simulink subsystem "Leds"  (R2023b)
settings: Solver=VariableStepAuto  StartTime=0.0  StopTime=10.0  RelTol=1e-3
libraries: arduinolib x3
settings Model: Creator=Usuario_UMA  LastModifiedBy=Felix

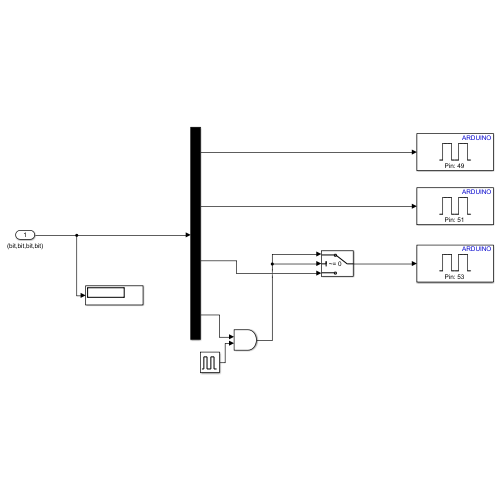
[thumbnail: Simulink's stored preview of the top-level diagram]
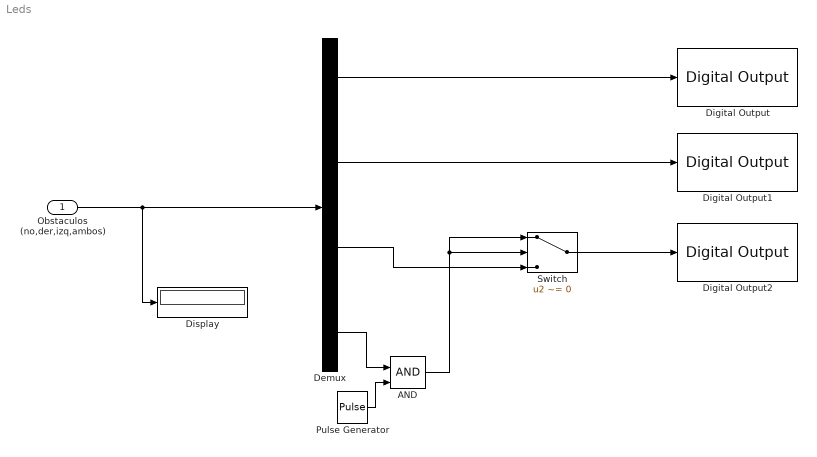
== system Leds ==
  Obstaculos (no,der,izq,ambos) : Inport
  AND : Logic  IconShape=distinctive  AllPortsSameDT=off  OutDataTypeStr=boolean
  Demux : Demux
  Digital Output : arduinolib/Digital Output  pinNumber=51  Direction=output  blockPlatform=arduino
  Digital Output1 : arduinolib/Digital Output  pinNumber=53  Direction=output  blockPlatform=arduino
  Digital Output2 : arduinolib/Digital Output  pinNumber=49  Direction=output  blockPlatform=arduino
  Display : Display
  Pulse Generator : DiscretePulseGenerator  PulseType=Time based  PulseWidth=5
  Switch : Switch  Criteria=u2 ~= 0  SaturateOnIntegerOverflow=off  InputSameDT=off
  wires:
  Demux/4 -> AND/1
  Demux/1 -> Digital Output/1
  Demux/2 -> Digital Output1/1
  Obstaculos (no,der,izq,ambos)/1 -> Demux/1, Display/1
  Pulse Generator/1 -> AND/2
  Switch/1 -> Digital Output2/1
  AND/1 -> Switch/1, Switch/2
  Demux/3 -> Switch/3
